simulink model "Dynamics_test_sim"  (R2016b)
settings: Solver=FixedStepAuto  StartTime=0.0  StopTime=1000  FixedStep=1  RelTol=1e-3
values from neighbouring files (symbols this model uses):
  init_accel = [0,0,20]    [Dynamics_test.m]
  init_pos = [1,1,-1]    [Dynamics_test.m]
  init_vel = [1,0,2]    [Dynamics_test.m]
  torque_init_const = [0,0,0]    [Dynamics_test.m]
undefined symbols (not defined in the file or in its folder): env_acc_eci_mps2, GPS_time, init_pos_eci_km, init_vel_eci_kmps, mag_vec_eci, sun_vec_eci
libraries: dynamics_lib x1, bus_stubs_template x1
settings Model: Creator=Ryan  LastModifiedBy=evich

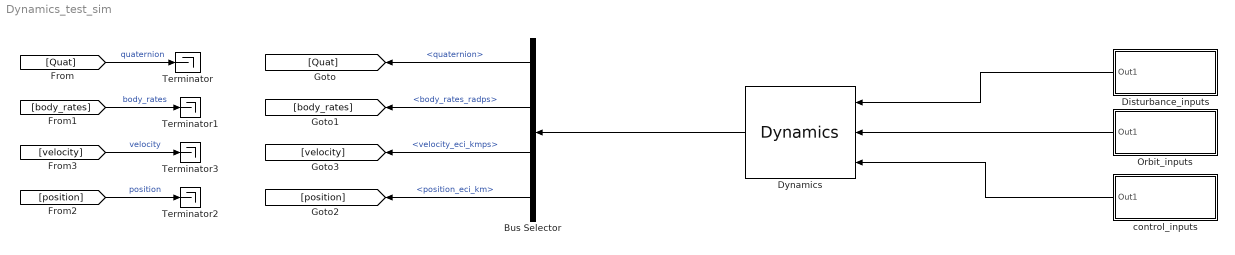
== system Dynamics_test_sim ==
  Bus Selector : BusSelector  OutputSignals=quaternion,body_rates_radps,velocity_eci_kmps,position_eci_km
  Disturbance_inputs : Subsystem
  Dynamics : dynamics_lib/Dynamics
  Orbit_inputs : Subsystem
  Terminator{,1..3} (4 alike) : Terminator
  control_inputs : Subsystem
  wires:
  control_inputs/1(Out1) -> Dynamics/3
  Disturbance_inputs/1(Out1) -> Dynamics/1
  Orbit_inputs/1(Out1) -> Dynamics/2
  Dynamics/1 -> Bus Selector/1
  Bus Selector/4 -> [position]  "<position_eci_km>"
  Bus Selector/3 -> [velocity]  "<velocity_eci_kmps>"
  Bus Selector/2 -> [body_rates]  "<body_rates_radps>"
  Bus Selector/1 -> [Quat]  "<quaternion>"
  [velocity] -> Terminator3/1  "velocity"
  [position] -> Terminator2/1  "position"
  [body_rates] -> Terminator1/1  "body_rates"
  [Quat] -> Terminator/1  "quaternion"

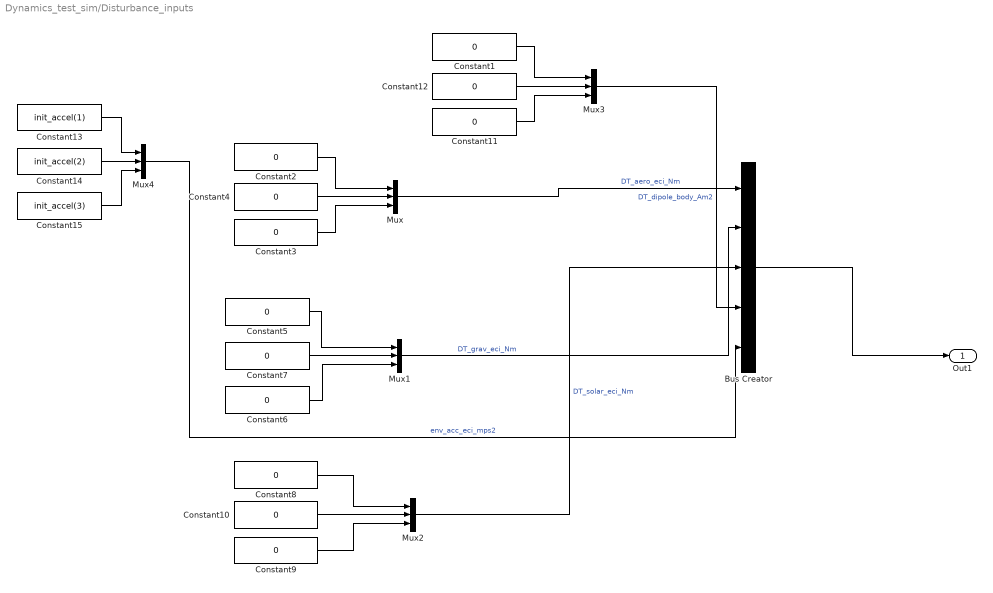
== system Dynamics_test_sim/Disturbance_inputs ==
  Bus Creator : BusCreator  Inputs=5
  Constant{1..12} (12 alike) : Constant  Value=0
  Constant13 : Constant  Value=init_accel(1)
  Constant14 : Constant  Value=init_accel(2)
  Constant15 : Constant  Value=init_accel(3)
  Mux{,1..4} (5 alike) : Mux  Inputs=3
  Out1 : Outport
  wires:
  Bus Creator/1 -> Out1/1
  Constant3/1 -> Mux/3
  Constant2/1 -> Mux/1
  Constant4/1 -> Mux/2
  Constant6/1 -> Mux1/3
  Constant5/1 -> Mux1/1
  Constant7/1 -> Mux1/2
  Constant9/1 -> Mux2/3
  Constant8/1 -> Mux2/1
  Constant10/1 -> Mux2/2
  Mux1/1 -> Bus Creator/2  "DT_grav_eci_Nm"
  Mux/1 -> Bus Creator/1  "DT_aero_eci_Nm"
  Mux2/1 -> Bus Creator/3  "DT_solar_eci_Nm"
  Constant11/1 -> Mux3/3
  Constant1/1 -> Mux3/1
  Constant12/1 -> Mux3/2
  Mux3/1 -> Bus Creator/4  "DT_dipole_body_Am2"
  Mux4/1 -> Bus Creator/5  "env_acc_eci_mps2"
  Constant14/1 -> Mux4/2
  Constant13/1 -> Mux4/1
  Constant15/1 -> Mux4/3

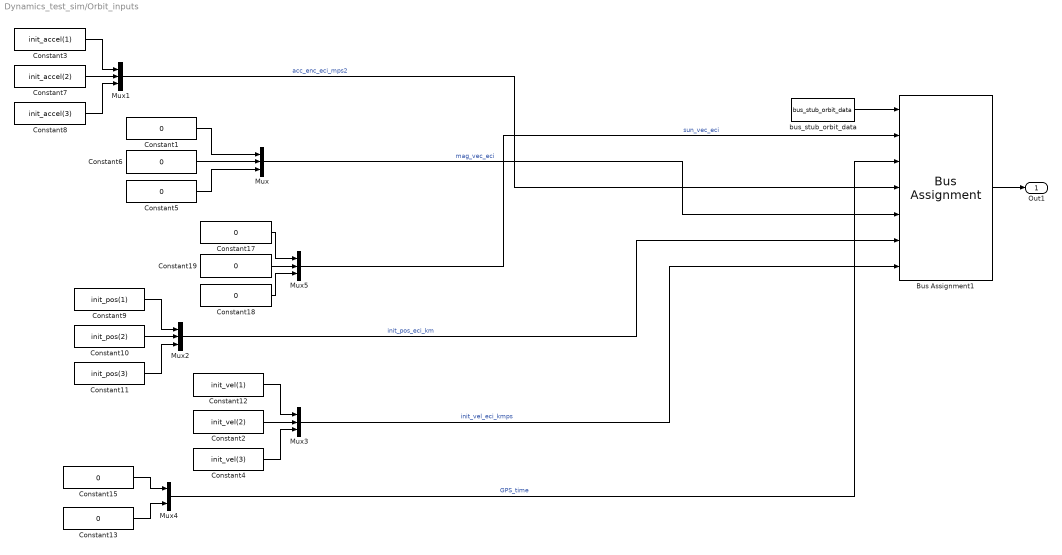
== system Dynamics_test_sim/Orbit_inputs ==
  Bus Assignment1 : BusAssignment  AssignedSignals=sun_vec_eci,GPS_time,env_acc_eci_mps2,mag_vec_eci,init_pos_eci_km,init_vel_eci_kmps
  Constant{1,5..6,13,15,17..19} (8 alike) : Constant  Value=0
  Constant10 : Constant  Value=init_pos(2)
  Constant11 : Constant  Value=init_pos(3)
  Constant12 : Constant  Value=init_vel(1)
  Constant2 : Constant  Value=init_vel(2)
  Constant3 : Constant  Value=init_accel(1)
  Constant4 : Constant  Value=init_vel(3)
  Constant7 : Constant  Value=init_accel(2)
  Constant8 : Constant  Value=init_accel(3)
  Constant9 : Constant  Value=init_pos(1)
  Mux{,1..3,5} (5 alike) : Mux  Inputs=3
  Mux4 : Mux  Inputs=2
  bus_stub_orbit_data : bus_stubs_template/bus_stub_orbit_data
  Out1 : Outport
  wires:
  Constant5/1 -> Mux/3
  Constant1/1 -> Mux/1
  Constant6/1 -> Mux/2
  Mux/1 -> Bus Assignment1/5  "mag_vec_eci"
  Mux1/1 -> Bus Assignment1/4  "acc_enc_eci_mps2"
  Mux3/1 -> Bus Assignment1/7  "init_vel_eci_kmps"
  Mux2/1 -> Bus Assignment1/6  "init_pos_eci_km"
  Constant7/1 -> Mux1/2
  Constant3/1 -> Mux1/1
  Constant8/1 -> Mux1/3
  Constant10/1 -> Mux2/2
  Constant9/1 -> Mux2/1
  Constant11/1 -> Mux2/3
  Constant2/1 -> Mux3/2
  Constant12/1 -> Mux3/1
  Constant4/1 -> Mux3/3
  Constant18/1 -> Mux5/3
  Constant17/1 -> Mux5/1
  Constant19/1 -> Mux5/2
  Mux4/1 -> Bus Assignment1/3  "GPS_time"
  Constant15/1 -> Mux4/1
  Constant13/1 -> Mux4/2
  bus_stub_orbit_data/1 -> Bus Assignment1/1
  Bus Assignment1/1 -> Out1/1
  Mux5/1 -> Bus Assignment1/2  "sun_vec_eci"

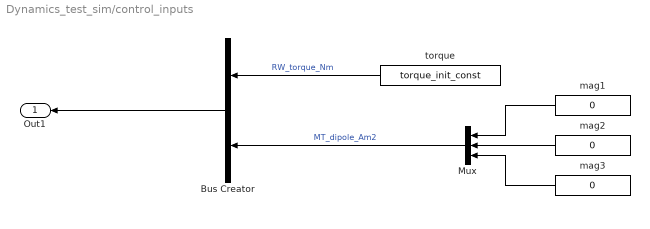
== system Dynamics_test_sim/control_inputs ==
  Bus Creator : BusCreator  Inputs=2
  Mux : Mux  Inputs=3
  mag1 : Constant  Value=0
  mag2 : Constant  Value=0
  mag3 : Constant  Value=0
  torque : Constant  Value=torque_init_const
  Out1 : Outport
  wires:
  mag1/1 -> Mux/1
  mag2/1 -> Mux/2
  mag3/1 -> Mux/3
  torque/1 -> Bus Creator/1  "RW_torque_Nm"
  Mux/1 -> Bus Creator/2  "MT_dipole_Am2"
  Bus Creator/1 -> Out1/1
